simulink model "speedgoat_IO397_Comms"  (R2022b)
settings: Solver=FixedStepDiscrete  StartTime=0.0  StopTime=inf  RelTol=1e-3
PreLoadFcn:
  | Ts = 0.001;
  | FPGA_Frequency = 75000000;
undefined symbols (not defined in the file): IO397
libraries: simulink x6, speedgoatlib_fpga x6, speedgoatlib_fpga_serial x3, speedgoatlib_fpga_analog_io x2, speedgoatlib_fpga_spi x2, hdlsllib x2
settings Model: SimulationMode=external  Creator=simon.beck  LastModifiedBy=jeffrey.gruenig
settings SolverCC: ConcurrentTasks=on  PositivePriorityOrder=on  MaxZcPerStep=1
settings DataIOCC: SaveFormat=StructureWithTime
settings OptimizationCC: BlockReduction=off  OptimizeBlockIOStorage=off  BufferReuse=off
settings DebuggingCC: UnderspecifiedInitializationDetection=Classic  MergeDetectMultiDrivingBlocksExec=none  TasksWithSamePriorityMsg=none
settings HardwareCC: ProdBitPerLong=64  ProdLongLongMode=on  ProdHWDeviceType=Intel->x86-64 (Linux 64)
settings ModelReferenceCC: EnableRefExpFcnMdlSchedulingChecks=on  PropagateSignalLabelsOutOfModel=off
settings RTWCC: Description=Simulink Real-Time  SystemTargetFile=slrealtime.tlc  TemplateMakefile=slrealtime_default_tmf  Toolchain=Simulink Real-Time Toolchain  BuildConfiguration=Faster Runs  CodeExecutionProfiling=on  TargetLang=C++  DLArmComputeVersion=19.05

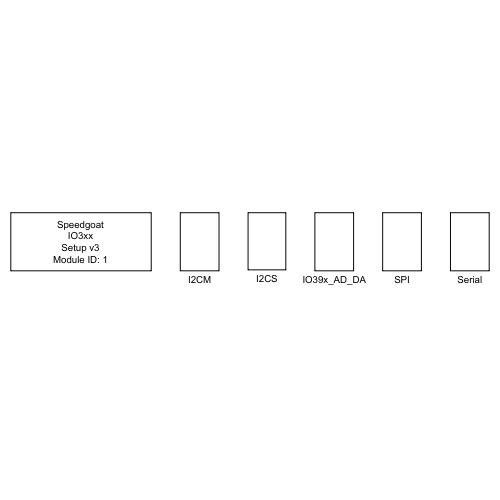
[thumbnail: Simulink's stored preview of the top-level diagram]
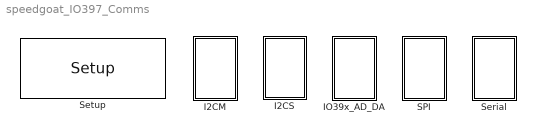
== system speedgoat_IO397_Comms ==
  I2CM : Subsystem
  I2CS : Subsystem
  IO39x_AD_DA : Subsystem
  SPI : Subsystem  Priority=1
  Serial : Subsystem
  Setup : speedgoatlib_fpga/Setup/Setup  board=IO397-50k  id=1  device_id=1  frontIO=None  rearIO=None  bitstreamFile=speedgoat_IO397_Comms.mat  rev=6.100000  timestamp_string=07/09/23 10:31:49  fpgaFreq=75 MHz  fpgaTick=13.33 ns  ProgSpiFlash=off  ProgBPIFlash=off  pciSlot=-1  useFpgaDmaController=off  PullRPort0=pull-up 3.3V  VioPort0=3.3V  PullRPort1=pull-up 3.3V  VioPort1=3.3V  PullRPort2=pull-up 3.3V  VioPort2=3.3V  PullRPort3=pull-up 3.3V  VioPort3=3.3V  PullRPort4=pull-up 3.3V  VioPort4=3.3V  PullRPort5=pull-up 3.3V  VioPort5=3.3V  PullRPort6=pull-up 3.3V  VioPort6=3.3V  diffLineTermination_rear1=on  diffLineTermination_rear2=on  diffLineTermination_rear3=on  diffLineTermination_rear4=on  diffLineTermination_rear5=on  diffLineTermination_rear6=on  diffLineTermination_rear7=on  diffLineTermination_rear8=on  PullRPort15=pull-up 3.3V  PullRPort31=pull-up 3.3V  PullRPort47=pull-up 3.3V  PullRPort63=pull-up 3.3V  diffLineTermination_1=on  diffLineTermination_2=on  diffLineTermination_3=on  diffLineTermination_4=on  diffLineTermination_5=on  diffLineTermination_6=on  diffLineTermination_7=on  diffLineTermination_8=on  diffLineTermination_9=on  diffLineTermination_10=on  diffLineTermination_11=on  diffLineTermination_12=on  diffLineTermination_13=on  diffLineTermination_14=on  diffLineTermination_15=on  diffLineTermination_16=on  diffLineTermination_17=on  diffLineTermination_18=on  diffLineTermination_19=on  diffLineTermination_20=on  diffLineTermination_21=on  diffLineTermination_22=on  diffLineTermination_23=on  diffLineTermination_24=on  diffLineTermination_25=on  diffLineTermination_26=on  diffLineTermination_27=on  diffLineTermination_28=on  diffLineTermination_29=on  diffLineTermination_30=on  diffLineTermination_31=on  diffLineTermination_32=on  Vo_36x_1=3.3V  Vi_Pull_36x_1=Floating  Vo_36x_2=3.3V  Vi_Pull_36x_2=Floating  Vo_36x_3=3.3V  Vi_Pull_36x_3=Floating  Vo_36x_4=3.3V  Vi_Pull_36x_4=Floating  Vo_36x_5=3.3V  Vi_Pull_36x_5=Floating  Vo_36x_6=3.3V  Vi_Pull_36x_6=Floating  Vo_36x_7=3.3V  Vi_Pull_36x_7=Floating  Vo_36x_8=3.3V  Vi_Pull_36x_8=Floating  Vo_36x_9_16=3.3V  Vi_Pull_36x_9_16=Floating  Vo_36x_17_24=3.3V  Vi_Pull_36x_17_24=Floating  Vo_36x_25_32=3.3V  Vi_Pull_36x_25_32=Floating  Vo_36x_33_40=3.3V  Vi_Pull_36x_33_40=Floating  Vo_36x_41_48=3.3V  Vi_Pull_36x_41_48=Floating  Vo_36x_49_56=3.3V  Vi_Pull_36x_49_56=Floating  Vo_36x_57_64=3.3V  Vi_Pull_36x_57_64=Floating
      settings: SourceProductName=Simulink Real-Time: Speedgoat I/O Blockset

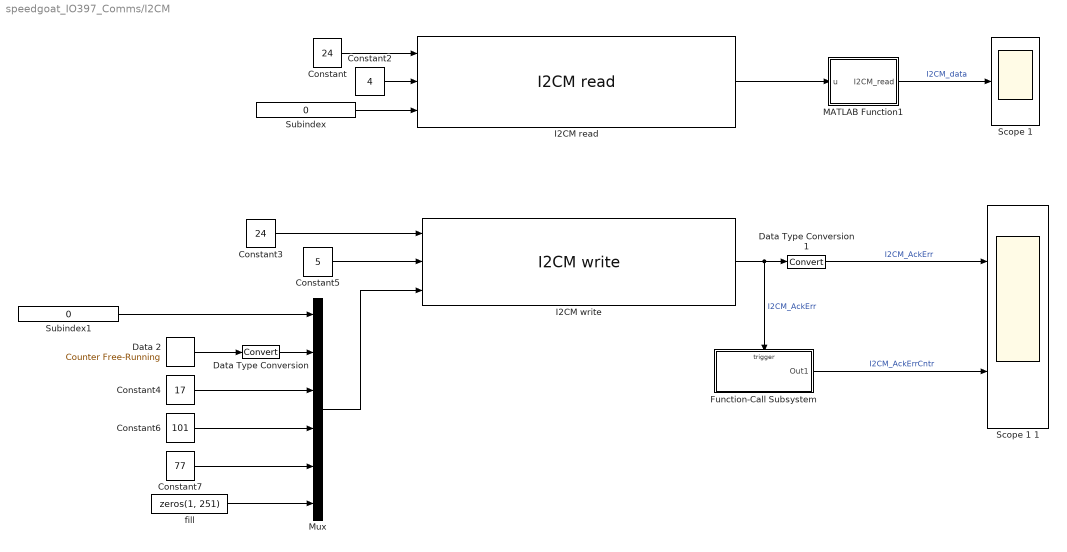
== system speedgoat_IO397_Comms/I2CM ==
  Constant : Constant  Value=24
  Constant2 : Constant  Value=4
  Constant3 : Constant  Value=24
  Constant4 : Constant  Value=17
  Constant5 : Constant  Value=5
  Constant6 : Constant  Value=101
  Constant7 : Constant  Value=77
  Data 2 : simulink/Sources/Counter Free-Running  NumBits=8  tsamp=-1
  Data Type Conversion : DataTypeConversion  SaturateOnIntegerOverflow=off  RndMeth=Floor
  Data Type Conversion1 : DataTypeConversion  SaturateOnIntegerOverflow=off  RndMeth=Floor
  Function-Call Subsystem : Subsystem  TreatAsAtomicUnit=on
  I2CM read : speedgoatlib_fpga/I2C/I2CM read  id=1  chan=1  ts=Ts*3  clockDivider=FPGA_Frequency/100e3/2  readPrevValue=off  subIndexConfiguration=on  showAckErrorPort=off
      settings: SourceProductName=Simulink Real-Time: Speedgoat I/O Blockset
  I2CM write : speedgoatlib_fpga/I2C/I2CM write  id=1  chan=1  ts=Ts*3  clockDivider=FPGA_Frequency/100e3/2  showAckErrorPort=on  readPrevValue=off
      settings: SourceProductName=Simulink Real-Time: Speedgoat I/O Blockset
  MATLAB Function1 : MATLAB Function  TreatAsAtomicUnit=on
  Mux : Mux  Inputs=6
  "Scope 1 " : Scope
  Scope 1 1 : Scope  NumInputPorts=2
  Subindex : Constant  Value=0
  Subindex1 : Constant  Value=0
  fill : Constant  Value=zeros(1, 251)
  wires:
  Data Type Conversion1/1 -> Scope 1 1/1  "I2CM_AckErr"
  Function-Call Subsystem/1(Out1) -> Scope 1 1/2  "I2CM_AckErrCntr"
  I2CM write/1 -> Function-Call Subsystem/Trigger, Data Type Conversion1/1  "I2CM_AckErr"
  Constant2/1 -> I2CM read/2
  Constant/1 -> I2CM read/1
  MATLAB Function1/1(I2CM_read) -> "Scope 1 "/1  "I2CM_data"
  I2CM read/1 -> MATLAB Function1/1(u)
  Subindex/1 -> I2CM read/3
  Mux/1 -> I2CM write/3
  fill/1 -> Mux/6
  Data Type Conversion/1 -> Mux/2
  Data 2/1 -> Data Type Conversion/1
  Constant5/1 -> I2CM write/2
  Constant3/1 -> I2CM write/1
  Constant4/1 -> Mux/3
  Constant6/1 -> Mux/4
  Constant7/1 -> Mux/5
  Subindex1/1 -> Mux/1

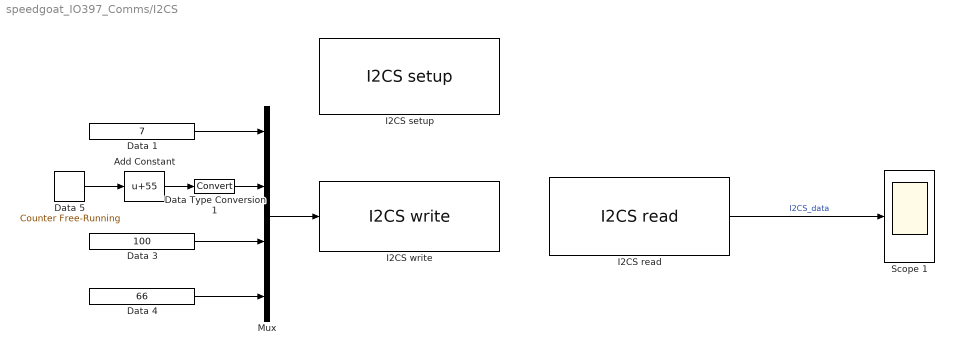
== system speedgoat_IO397_Comms/I2CS ==
  Add Constant : Bias  Bias=55  SaturateOnIntegerOverflow=off
  Data 1 : Constant  Value=7
  Data 3 : Constant  Value=100
  Data 4 : Constant  Value=66
  Data 5 : simulink/Sources/Counter Free-Running  NumBits=8  tsamp=-1
  Data Type Conversion1 : DataTypeConversion  SaturateOnIntegerOverflow=off  RndMeth=Floor
  I2CS read : speedgoatlib_fpga/I2C/I2CS read  id=1  chan=[1]  regs=[1,2,3,4]  ts=Ts*3  showDataValidPort=off  showLastRegPort=off  showLastRegValidPort=off
      settings: SourceProductName=Simulink Real-Time: Speedgoat I/O Blockset
  I2CS setup : speedgoatlib_fpga/I2C/I2CS setup  id=1  chan=[1]  slaveID=[24]  skipRegAddress=off  ts=-1
      settings: SourceProductName=Simulink Real-Time: Speedgoat I/O Blockset
  I2CS write : speedgoatlib_fpga/I2C/I2CS write  id=1  chan=[1]  regs=[1, 2, 3, 4]  ts=Ts*3
      settings: SourceProductName=Simulink Real-Time: Speedgoat I/O Blockset
  Mux : Mux
  "Scope 1 " : Scope
  wires:
  Mux/1 -> I2CS write/1
  I2CS read/1 -> "Scope 1 "/1  "I2CS_data"
  Data 4/1 -> Mux/4
  Data 3/1 -> Mux/3
  Data Type Conversion1/1 -> Mux/2
  Data 5/1 -> Add Constant/1
  Data 1/1 -> Mux/1
  Add Constant/1 -> Data Type Conversion1/1

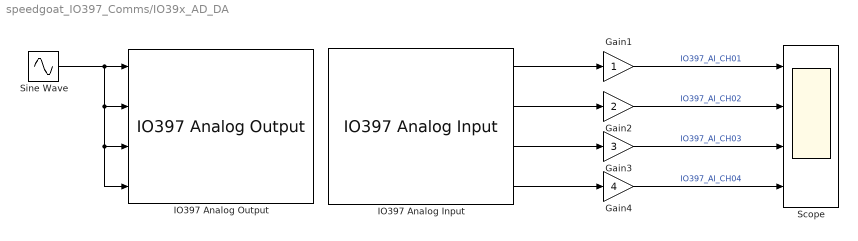
== system speedgoat_IO397_Comms/IO39x_AD_DA ==
  Gain1 : Gain
  Gain2 : Gain  Gain=2
  Gain3 : Gain  Gain=3
  Gain4 : Gain  Gain=4
  IO397 Analog Input : speedgoatlib_fpga_analog_io/IO397 Analog Input  openMaskCallback=0  id=1  chan=[1:4]  range=+-5 V  parAiTriggerMode=I/O Module Clock  parAiInternalSignal=None  parAiDioTriggerChannel=1  parAiSampleRate=0  trigger=Initiator  ts=0.001
      settings: SourceProductName=Simulink Real-Time: Speedgoat I/O Blockset
  IO397 Analog Output : speedgoatlib_fpga_analog_io/IO397 Analog Output  id=1  chan=1:4  initVal=0  resetVal=0  ts=0.001  span=+-5 V
      settings: SourceProductName=Simulink Real-Time: Speedgoat I/O Blockset
  Scope : Scope  NumInputPorts=4
  Sine Wave : Sin  Frequency=2*pi*(1/Ts)/50  SampleTime=Ts
  wires:
  IO397 Analog Input/4 -> Gain4/1
  IO397 Analog Input/3 -> Gain3/1
  IO397 Analog Input/2 -> Gain2/1
  IO397 Analog Input/1 -> Gain1/1
  Gain4/1 -> Scope/4  "IO397_AI_CH04"
  Gain3/1 -> Scope/3  "IO397_AI_CH03"
  Gain2/1 -> Scope/2  "IO397_AI_CH02"
  Gain1/1 -> Scope/1  "IO397_AI_CH01"
  Sine Wave/1 -> IO397 Analog Output/1, IO397 Analog Output/3, IO397 Analog Output/4, IO397 Analog Output/2

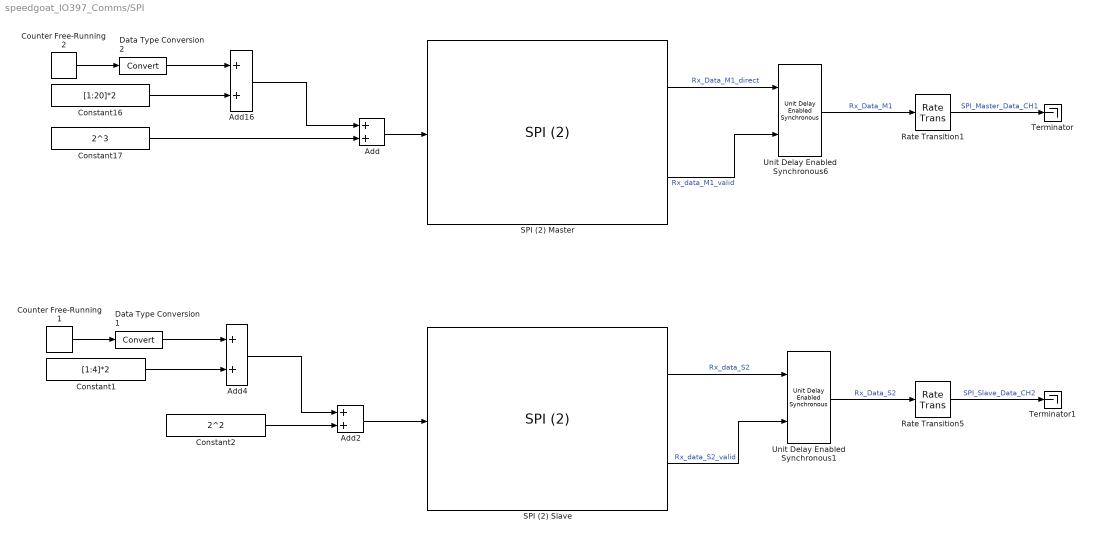
== system speedgoat_IO397_Comms/SPI ==
  Add : Sum  OutDataTypeStr=Inherit: Inherit via back propagation  InputSameDT=on
  Add16 : Sum
  Add2 : Sum  OutDataTypeStr=Inherit: Inherit via back propagation  InputSameDT=on
  Add4 : Sum
  Constant1 : Constant  Value=[1:4]*2  OutDataTypeStr=Inherit: Inherit via back propagation
  Constant16 : Constant  Value=[1:20]*2  OutDataTypeStr=Inherit: Inherit via back propagation
  Constant17 : Constant  Value=2^3  OutDataTypeStr=Inherit: Inherit via back propagation
  Constant2 : Constant  Value=2^2  OutDataTypeStr=Inherit: Inherit via back propagation
  Counter Free-Running1 : simulink/Sources/Counter Free-Running  NumBits=32  tsamp=-1
  Counter Free-Running2 : simulink/Sources/Counter Free-Running  NumBits=32  tsamp=-1
  Data Type Conversion1 : DataTypeConversion  SaturateOnIntegerOverflow=off  RndMeth=Floor
  Data Type Conversion2 : DataTypeConversion  SaturateOnIntegerOverflow=off  RndMeth=Floor
  Rate Transition1 : RateTransition  Deterministic=off
  Rate Transition5 : RateTransition  Deterministic=off
  SPI (2) Master : speedgoatlib_fpga_spi/SPI (2)  Priority=1  id=1  chan=[1]  samp_time=Ts*7  board=IO397-50k  pciSlot=-1  role=Master  sync_mode=off  multislave_mode=off  write_only=off  read_only=off  enableDma=off  multislave_chan=[1:8]  cpol=[0]  cpha=[1]  frequency=[2e6]  frequency_eff=1.974e6  delay_start=[2e-6]  delay_start_eff=2e-6  delay_interword=[2e-6]  delay_interword_eff=2e-6  delay_stop=[2e-6]  delay_stop_eff=2e-6  delay_compensation=[100e-9]  delay_compensation_eff=106.7e-9  words_per_frame=[20]  dynamic_words_per_frame=off  bits_per_word=[20]  bit_shift_lsb_first=[0]  no_cs=off  clock_timeout=[1e-6]  clock_timeout_eff=1E-06
      settings: SourceProductName=Simulink Real-Time: Speedgoat I/O Blockset
  SPI (2) Slave : speedgoatlib_fpga_spi/SPI (2)  id=1  chan=[2]  samp_time=Ts*20  board=IO397-50k  pciSlot=-1  role=Slave  sync_mode=on  multislave_mode=off  write_only=off  read_only=off  enableDma=off  multislave_chan=[1]  cpol=[0]  cpha=[1]  frequency=[100e3]  frequency_eff=100000  delay_start=[1e-6]  delay_start_eff=1.06667E-07  delay_interword=[1e-6]  delay_interword_eff=1E-06  delay_stop=[1e-6]  delay_stop_eff=1E-06  delay_compensation=[1e-6]  delay_compensation_eff=1E-06  words_per_frame=[4]  dynamic_words_per_frame=off  bits_per_word=[20]  bit_shift_lsb_first=[0]  no_cs=off  clock_timeout=[10e-6]  clock_timeout_eff=1E-06
      settings: SourceProductName=Simulink Real-Time: Speedgoat I/O Blockset
  Terminator : Terminator
  Terminator1 : Terminator
  Unit Delay Enabled Synchronous1 : hdlsllib/Discrete/Unit Delay Enabled Synchronous  InitialCondition=0.0  SampleTime=-1
  Unit Delay Enabled Synchronous6 : hdlsllib/Discrete/Unit Delay Enabled Synchronous  InitialCondition=0.0  SampleTime=-1
  wires:
  Data Type Conversion1/1 -> Add4/1
  Constant16/1 -> Add16/2
  SPI (2) Master/1 -> Unit Delay Enabled Synchronous6/1  "Rx_Data_M1_direct"
  Counter Free-Running2/1 -> Data Type Conversion2/1
  Rate Transition5/1 -> Terminator1/1  "SPI_Slave_Data_CH2"
  Data Type Conversion2/1 -> Add16/1
  Unit Delay Enabled Synchronous1/1 -> Rate Transition5/1  "Rx_Data_S2"
  Constant1/1 -> Add4/2
  Rate Transition1/1 -> Terminator/1  "SPI_Master_Data_CH1"
  Unit Delay Enabled Synchronous6/1 -> Rate Transition1/1  "Rx_Data_M1"
  SPI (2) Master/2 -> Unit Delay Enabled Synchronous6/2  "Rx_data_M1_valid"
  SPI (2) Slave/2 -> Unit Delay Enabled Synchronous1/2  "Rx_data_S2_valid"
  Constant17/1 -> Add/2
  Add16/1 -> Add/1
  Counter Free-Running1/1 -> Data Type Conversion1/1
  Add4/1 -> Add2/1
  SPI (2) Slave/1 -> Unit Delay Enabled Synchronous1/1  "Rx_data_S2"
  Constant2/1 -> Add2/2
  Add/1 -> SPI (2) Master/1
  Add2/1 -> SPI (2) Slave/1

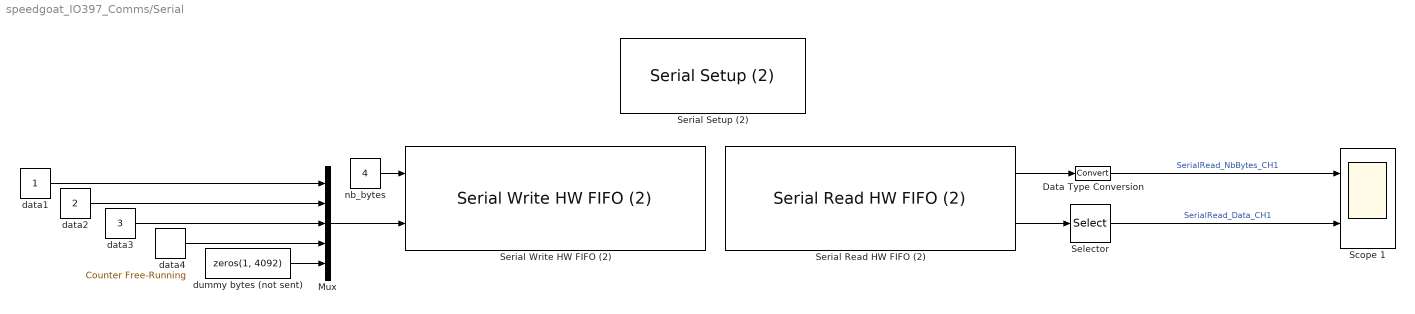
== system speedgoat_IO397_Comms/Serial ==
  Data Type Conversion : DataTypeConversion  SaturateOnIntegerOverflow=off  RndMeth=Floor
  Mux : Mux  Inputs=5
  "Scope 1 " : Scope  NumInputPorts=2
  Selector : Selector  InputPortWidth=4096  IndexOptions=Index vector (dialog)  Indices=1:4  OutputSizes=1
  Serial Read HW FIFO (2) : speedgoatlib_fpga_serial/Serial Read HW FIFO (2)  id=1  channel=1  board=IO397-50k  pciSlot=-1  ts=0.001  data_length=8
      settings: SourceProductName=Simulink Real-Time: Speedgoat I/O Blockset
  Serial Setup (2) : speedgoatlib_fpga_serial/Serial Setup (2)  id=1  channel=[1]  bitrate=[1e6]  bitrate_effective=986.8421e3  bitrate_error=-1.3158  parity_mode=No parity  data_length=[8]  stop_length=[2]  enable_half_duplex=[0]  rx_character_timeout=[0]  board=IO397-50k  pciSlot=-1
      settings: SourceProductName=Simulink Real-Time: Speedgoat I/O Blockset
  Serial Write HW FIFO (2) : speedgoatlib_fpga_serial/Serial Write HW FIFO (2)  id=1  channel=1  board=IO397-50k  pciSlot=-1  ts=0.001  data_length=8
      settings: SourceProductName=Simulink Real-Time: Speedgoat I/O Blockset
  data1 : Constant  OutDataTypeStr=Inherit: Inherit via back propagation
  data2 : Constant  Value=2  OutDataTypeStr=Inherit: Inherit via back propagation
  data3 : Constant  Value=3  OutDataTypeStr=Inherit: Inherit via back propagation
  data4 : simulink/Sources/Counter Free-Running  NumBits=8  tsamp=-1
  dummy bytes (not sent) : Constant  Value=zeros(1, 4092)  OutDataTypeStr=Inherit: Inherit via back propagation
  nb_bytes : Constant  Value=4  OutDataTypeStr=Inherit: Inherit via back propagation
  wires:
  Selector/1 -> "Scope 1 "/2  "SerialRead_Data_CH1"
  Data Type Conversion/1 -> "Scope 1 "/1  "SerialRead_NbBytes_CH1"
  data1/1 -> Mux/1
  nb_bytes/1 -> Serial Write HW FIFO (2)/1
  Serial Read HW FIFO (2)/2 -> Selector/1
  dummy bytes (not sent)/1 -> Mux/5
  Mux/1 -> Serial Write HW FIFO (2)/2
  data2/1 -> Mux/2
  Serial Read HW FIFO (2)/1 -> Data Type Conversion/1
  data3/1 -> Mux/3
  data4/1 -> Mux/4

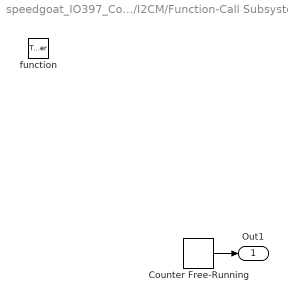
== system speedgoat_IO397_Comms/I2CM/Function-Call Subsystem ==
  function : TriggerPort  VariantControl=(inherit)
  Counter Free-Running : simulink/Sources/Counter Free-Running  NumBits=32  tsamp=-1
  Out1 : Outport
  wires:
  Counter Free-Running/1 -> Out1/1

== matlab function speedgoat_IO397_Comms/I2CM/MATLAB Function1 ==
  data: u input; I2CM_read output
function I2CM_read = fcn(u)
%#codegen

I2CM_read = [ u(1), u(2), u(3), u(4)];
